simulink model "toy_model_NO1"  (R2015a)
settings: Solver=FixedStepDiscrete  SolverMode=SingleTasking  StartTime=0  StopTime=10  FixedStep=0.001024  RelTol=1e-3
PostLoadFcn:
  | mdm_postload_callback(gcs);
model workspace (MAT data in the model file):
  autoc_mdd_data01 : struct (value not decoded)
PreSaveFcn:
  | %mdm_presave_callback(gcs);
CloseFcn:
  | mdm_close_callback(gcs);
Description:
  | AutoCodeGenerator:Version 1.05.A;
settings Model: autoc_dsminitmode=spec  autoc_cdm_savetype=ModelWorkspace  autoc_cdm_name=autoc_mdd_data01  autoc_current_model=toy_model_NO1  VCB_Name=no Correction Bundle  VCB_Version=-  VCB_Release=R2010b  VCB_Date=10-Oct-2013  VCB_SPver=Service Pack 2  ExtModeTrigMode=oneshot  ExtModeArmWhenConnect=off  Creator=E2XR 1G OKA  LastModifiedBy=xjin
settings DataIOCC: LimitDataPoints=off  SignalLoggingSaveFormat=ModelDataLogs
settings OptimizationCC: InlineParams=on  UseDivisionForNetSlopeComputation=UseDivisionForReciprocalsOfIntegersOnly  UseSpecifiedMinMax=on  InlineInvariantSignals=on  EnhancedBackFolding=on  StrengthReduction=on  EnableMemcpy=off  PassReuseOutputArgsAs=Individual arguments  ExpressionDepthLimit=2147483647  ZeroExternalMemoryAtStartup=off  ZeroInternalMemoryAtStartup=off  InitFltsAndDblsToZero=on  NoFixptDivByZeroProtection=on  EfficientFloat2IntCast=on  OptimizeModelRefInitCode=on  LifeSpan=1
settings DebuggingCC: ConsistencyChecking=warning  SignalInfNanChecking=warning  SignalRangeChecking=warning  AlgebraicLoopMsg=error  UnderspecifiedInitializationDetection=Classic  CheckExecutionContextPreStartOutputMsg=on  CheckExecutionContextRuntimeOutputMsg=on  TimeAdjustmentMsg=warning  InheritedTsInSrcMsg=none  MultiTaskDSMMsg=warning  MultiTaskCondExecSysMsg=none  SingleTaskRateTransMsg=warning  TasksWithSamePriorityMsg=none  SigSpecEnsureSampleTimeMsg=error  ParameterPrecisionLossMsg=none  ParameterTunabilityLossMsg=none  FixptConstUnderflowMsg=error  FixptConstOverflowMsg=error  FixptConstPrecisionLossMsg=warning  VectorMatrixConversionMsg=warning  FcnCallInpInsideContextMsg=UseLocalSettings  UnconnectedInputMsg=error  UnconnectedOutputMsg=error  UnconnectedLineMsg=error  UniqueDataStoreMsg=error  BusObjectLabelMismatch=error  RootOutportRequireBusObject=error  ModelReferenceIOMsg=warning  ModelReferenceVersionMismatchMessage=warning  ModelReferenceIOMismatchMessage=warning  StateNameClashWarn=warning  StrictBusMsg=ErrorOnBusTreatedAsVector  BusNameAdapt=ErrorWithoutRepair
settings HardwareCC: ProdIntDivRoundTo=Zero  ProdEndianess=LittleEndian  ProdHWDeviceType=NEC->V850  TargetHWDeviceType=32-bit Generic
settings ModelReferenceCC: UpdateModelReferenceTargets=IfOutOfDate
settings RTWCC: SystemTargetFile=ert_denso.tlc  GenCodeOnly=on  TemplateMakefile=ert_autoc.tmf  Description=Real-Time Workshop Embedded Coder  RTWVerbose=off
settings CodeAppCC: ForceParamTrailComments=on  IgnoreCustomStorageClasses=off  SFDataObjDesc=on  CustomSymbolStrType=$N$R$M  CustomSymbolStrFcnArg=rtu_$N$M  CustomSymbolStrBlkIO=_atctmp_rtb_$N$M  CustomSymbolStrTmpVar=_atctmp_rtb_$N$M  InsertBlockDesc=on  InternalIdentifier=Classic
settings ERTTargetCC: TargetFcnLib=ansi_tfl_tmw.mat  CodeReplacementLibrary=Auto-C FixedPoint Library  GenerateSampleERTMain=off  ParMdlRefBuildCompliant=on  CompOptLevelCompliant=on  ConcurrentExecutionCompliant=on  IncludeMdlTerminateFcn=off  SuppressErrorStatus=on  ERTFirstTimeCompliant=on  SupportAbsoluteTime=off  SupportNonFinite=off  SupportComplex=off  SupportContinuousTime=off  SupportVariableSizeSignals=off  ParenthesesLevel=Maximum  ModelStepFunctionPrototypeControlCompliant=on  CPPClassGenCompliant=on  ExtModeMexFile=noextcomm  RootIOFormat=Structure reference  ERTSrcFileBannerTemplate=code_c_template_cgt.tlc  ERTHdrFileBannerTemplate=code_h_template_cgt.tlc  ERTDataSrcFileTemplate=data_c_template_cgt.tlc  ERTDataHdrFileTemplate=data_h_template_cgt.tlc  ERTCustomFileTemplate=autoc_file_process_cgt.tlc  PreserveExpressionOrder=on  PreserveExternInFcnDecls=off  MemSecPackage=Simulink  MemSecDataConstants=MemConstVolatile

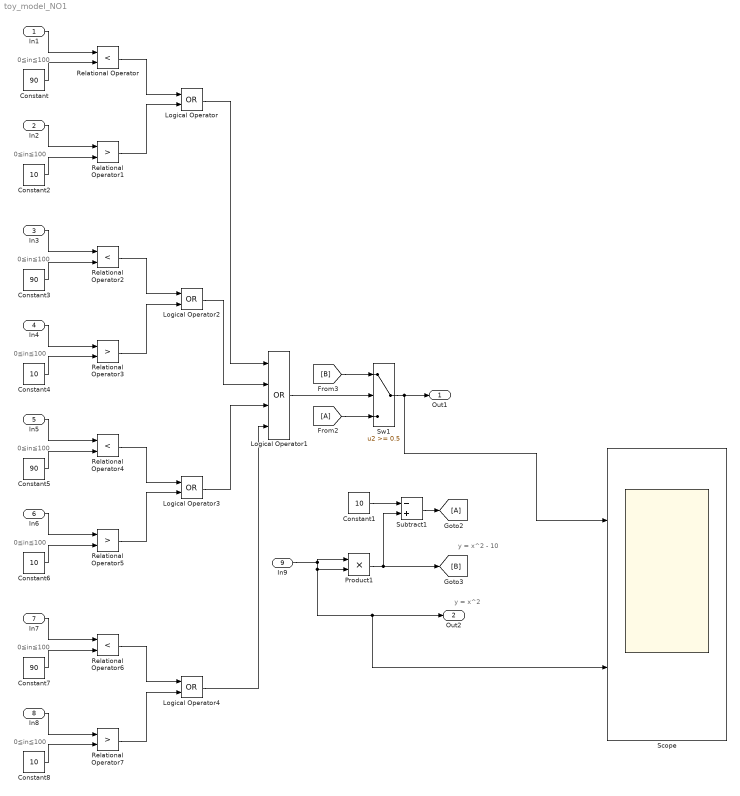
== system toy_model_NO1 ==
  note: 0≦in≦100
  note: 0≦in≦100
  note: 0≦in≦100
  note: 0≦in≦100
  note: 0≦in≦100
  note: 0≦in≦100
  note: 0≦in≦100
  note: 0≦in≦100
  note: y = x^2
  note: y = x^2 - 10
  In1 : Inport
  In2 : Inport  Port=2
  In3 : Inport  Port=3
  In4 : Inport  Port=4
  In5 : Inport  Port=5
  In6 : Inport  Port=6
  In7 : Inport  Port=7
  In8 : Inport  Port=8
  In9 : Inport  Port=9
  Constant{,3,5,7} (4 alike) : Constant  Value=90
  Constant{1..2,4,6,8} (5 alike) : Constant  Value=10
  Logical Operator{,2..4} (4 alike) : Logic  Operator=OR  AllPortsSameDT=off  OutDataTypeStr=boolean
  Logical Operator1 : Logic  Operator=OR  Inputs=4  AllPortsSameDT=off  OutDataTypeStr=boolean
  Product1 : Product  RndMeth=Zero
  Relational Operator{,2,4,6} (4 alike) : RelationalOperator  Operator=<  OutDataTypeStr=boolean
  Relational Operator{1,3,5,7} (4 alike) : RelationalOperator  Operator=>  OutDataTypeStr=boolean
  Scope : Scope  NumInputPorts=2
      settings: TimeRange=auto  MaxDataPoints=5000  SaveToWorkspace=off  SaveName=ScopeData  YMin=-5~-5  YMax=5~5  SampleTime=-1
  Subtract1 : Sum  Inputs=-+
  Sw1 : Switch  Threshold=0.5  RndMeth=Simplest  InputSameDT=on
  Out1 : Outport
  Out2 : Outport  Port=2
  wires:
  Logical Operator1/1 -> Sw1/2
  [B] -> Sw1/1
  [A] -> Sw1/3
  Product1/1 -> Subtract1/2, [B]
  Constant1/1 -> Subtract1/1
  Subtract1/1 -> [A]
  In1/1 -> Relational Operator/1
  Constant/1 -> Relational Operator/2
  In2/1 -> Relational Operator1/1
  Constant2/1 -> Relational Operator1/2
  Relational Operator/1 -> Logical Operator/1
  Relational Operator1/1 -> Logical Operator/2
  In3/1 -> Relational Operator2/1
  Constant3/1 -> Relational Operator2/2
  In4/1 -> Relational Operator3/1
  Constant4/1 -> Relational Operator3/2
  Relational Operator2/1 -> Logical Operator2/1
  Relational Operator3/1 -> Logical Operator2/2
  In5/1 -> Relational Operator4/1
  Constant5/1 -> Relational Operator4/2
  In6/1 -> Relational Operator5/1
  Constant6/1 -> Relational Operator5/2
  Relational Operator4/1 -> Logical Operator3/1
  Relational Operator5/1 -> Logical Operator3/2
  In7/1 -> Relational Operator6/1
  Constant7/1 -> Relational Operator6/2
  In8/1 -> Relational Operator7/1
  Constant8/1 -> Relational Operator7/2
  Relational Operator6/1 -> Logical Operator4/1
  Relational Operator7/1 -> Logical Operator4/2
  Logical Operator/1 -> Logical Operator1/1
  Logical Operator2/1 -> Logical Operator1/2
  Logical Operator3/1 -> Logical Operator1/3
  Logical Operator4/1 -> Logical Operator1/4
  Sw1/1 -> Scope/1, Out1/1
  In9/1 -> Product1/1, Product1/2, Scope/2, Out2/1
